simulink model "waypoint_generation_ptCloud_200802_mapdata_filtering_8m_2"  (R2020a)
settings: Solver=ode4  StartTime=0.0  StopTime=500  FixedStep=0.01  RelTol=1e-3  EnableMultiTasking=on
InitFcn:
  | detector = load('ptOPDetector.mat');
  | OPdetector = detector.OPdetector;
undefined symbols (not defined in the file): g, Kd_p, Kd_q, Kd_r, Kd_vx, Kd_vy, Kd_vz, Kff_r, Kff_vx, Kff_vy, Kff_vz, Ki_p, Ki_q, Ki_r, Ki_vx, Ki_vy, Ki_vz, Kp_p, Kp_phi, Kp_psi, Kp_q, Kp_r, Kp_theta, Kp_vx, Kp_vy, Kp_vz, M, pointCloud_center, sigma_motor, w_h
libraries: visiontextngfix x4, sharedtransform x1, shared6dof x1, simulink_extras x1
(part 2 of 3)

== matlab function waypoint_generation_ptCloud_200802_mapdata_filtering_8m_2/3D A* Algorithm/MATLAB Function2 ==
  data: current_pos input; point input; distance input; I_front_rgb input; I_back_rgb input; I_left_rgb input; I_right_rgb input; bboxes_front_raw input; openpoint_front output; bboxes_back_raw input; bboxes_left_raw input; bboxes_right_raw input; openpoint_back output; openpoint_left output; openpoint_right output; image_grid input; count output
function [openpoint_front,openpoint_back,openpoint_left,openpoint_right,count] = fcn(current_pos,point,distance,I_front_rgb,I_back_rgb,I_left_rgb,I_right_rgb,bboxes_front_raw,bboxes_back_raw,bboxes_left_raw,bboxes_right_raw,image_grid)
% function [distance_ref_front,distance_ref_back,distance_ref_left,distance_ref_right] = fcn(point,I_front_rgb,I_back_rgb,I_left_rgb,I_right_rgb,bboxes_front_raw,bboxes_back_raw,bboxes_left_raw,bboxes_right_raw)
% image_grid = 0.05;

pos_x = current_pos(1);
pos_y = current_pos(2);
pos_z = current_pos(3);

I_front = I_front_rgb(:,:,1);
I_back = I_back_rgb(:,:,1);
I_left = I_left_rgb(:,:,1);
I_right = I_right_rgb(:,:,1);

openpoint_front = nan(5,6);
openpoint_back = nan(5,6);
openpoint_left = nan(5,6);
openpoint_right = nan(5,6);
count = zeros(5,4);
thickness = distance/2;
% thickness = 2;

% bboxes_front = int16(nonzeros(bboxes_front_raw));
% bboxes_back = int16(nonzeros(bboxes_back_raw));
% bboxes_left = int16(nonzeros(bboxes_left_raw));
% bboxes_right = int16(nonzeros(bboxes_right_raw));
bboxes_front = int16(bboxes_front_raw);
bboxes_back = int16(bboxes_back_raw);
bboxes_left = int16(bboxes_left_raw);
bboxes_right = int16(bboxes_right_raw);
% distance_ref_front=[];
% distance_ref_back=[];
% distance_ref_left=[];
% distance_ref_right=[];

distance_ref_front=nan(5,1);
distance_ref_back=nan(5,1);
distance_ref_left=nan(5,1);
distance_ref_right=nan(5,1);

% aaa=1;
% if ~isempty(bboxes_front)
if ~sum(bboxes_front)==0
    for aaa = 1:numel(nonzeros(bboxes_front))/4
        if (bboxes_front(aaa,1)+bboxes_front(aaa,3)/2) >= length(I_front)/2
            distance_ref_front(aaa) = bboxes_front(aaa,1)+bboxes_front(aaa,3);
        else
            distance_ref_front(aaa) = bboxes_front(aaa,1);
        end
    end
    distance_ref_front= -(distance_ref_front - length(I_front)/2)*image_grid;           % 醫뚰몴媛?(m)
end

% if ~isempty(bboxes_back)
if ~sum(bboxes_back)==0
    for aaa = 1:numel(nonzeros(bboxes_back))/4
        if (bboxes_back(aaa,1)+bboxes_back(aaa,3)/2) >= length(I_back)/2
            distance_ref_back(aaa) = bboxes_back(aaa,1)+bboxes_back(aaa,3);
        else
            distance_ref_back(aaa) = bboxes_back(aaa,1);
        end
    end
    distance_ref_back= -(distance_ref_back - length(I_back)/2)*image_grid;              % 醫뚰몴媛?(m)
end

% if ~isempty(bboxes_left)
if ~sum(bboxes_left)==0
    for aaa = 1:numel(nonzeros(bboxes_left))/4
        if (bboxes_left(aaa,1)+bboxes_left(aaa,3)/2) >= length(I_left)/2
            distance_ref_left(aaa) = bboxes_left(aaa,1)+bboxes_left(aaa,3);
        else
            distance_ref_left(aaa) = bboxes_left(aaa,1);
        end
    end
    distance_ref_left= (distance_ref_left - length(I_left)/2)*image_grid;              % 醫뚰몴媛?(m)
end

% if ~isempty(bboxes_right)
if ~sum(bboxes_right)==0
    for aaa = 1:numel(nonzeros(bboxes_right))/4
        if (bboxes_right(aaa,1)+bboxes_right(aaa,3)/2) >= length(I_right)/2
            distance_ref_right(aaa) = bboxes_right(aaa,1)+bboxes_right(aaa,3);
        else
            distance_ref_right(aaa) = bboxes_right(aaa,1);
        end
    end
    distance_ref_right= (distance_ref_right - length(I_right)/2)*image_grid;            % 醫뚰몴媛?(m)
end

% scale = 5;
scale = 10;
distance_fb_max=-ones(length(distance_ref_front),1)*image_grid*length(I_front)/2;
distance_fb_min=ones(length(distance_ref_back),1)*image_grid*length(I_back)/2;
distance_lr_max=-ones(length(distance_ref_left),1)*image_grid*length(I_left)/2;
distance_lr_min=ones(length(distance_ref_right),1)*image_grid*length(I_right)/2;

% distance_fb_max=ones(5,1)*distance;
% distance_fb_min=-ones(5,1)*distance;
% distance_lr_max=ones(5,1)*distance;
% distance_lr_min=-ones(5,1)*distance;
    
for bbb=1:length(point)
    %     if ~isempty(distance_ref_front)
    for aaa = 1:length(distance_ref_front)
        if ~isnan(distance_ref_front(aaa))
            if point(bbb,2)>=(distance_ref_front(aaa)-image_grid*scale) && point(bbb,2)<=(distance_ref_front(aaa)+image_grid*scale)
                if point(bbb,1) > distance_fb_max(aaa)
                    distance_fb_max(aaa) = point(bbb,1);
                end
            end
        end
    end
    %     if ~isempty(distance_ref_back)
    for aaa = 1:length(distance_ref_back)
        if ~isnan(distance_ref_back(aaa))
            if point(bbb,2)>=(distance_ref_back(aaa)-image_grid*scale) && point(bbb,2)<=(distance_ref_back(aaa)+image_grid*scale)
                if point(bbb,1) < distance_fb_min(aaa)
                    distance_fb_min(aaa) = point(bbb,1);
                end
            end
        end
    end
    %     if ~isempty(distance_ref_left)
    for aaa = 1:length(distance_ref_left)
        if ~isnan(distance_ref_left(aaa))
            if point(bbb,1)>=(distance_ref_left(aaa)-image_grid*scale) && point(bbb,1)<=(distance_ref_left(aaa)+image_grid*scale)
                if point(bbb,2) > distance_lr_max(aaa)
                    distance_lr_max(aaa) = point(bbb,2);
                end
            end
        end
    end
    %     if ~isempty(distance_ref_right)
    for aaa = 1:length(distance_ref_right)
        if ~isnan(distance_ref_right(aaa))
            if point(bbb,1)>=(distance_ref_right(aaa)-image_grid*scale) && point(bbb,1)<=(distance_ref_right(aaa)+image_grid*scale)
                if point(bbb,2) < distance_lr_min(aaa)
                    distance_lr_min(aaa) = point(bbb,2);
                end
            end
        end
    end
end
bboxes_transformed_front = -(double(bboxes_front)-[ones(5,1)*length(I_front)/2, ones(5,1)*length(I_front)/2, zeros(5,1), zeros(5,1)])*image_grid;
bboxes_transformed_back = -(double(bboxes_back)-[ones(5,1)*length(I_back)/2, ones(5,1)*length(I_back)/2, zeros(5,1), zeros(5,1)])*image_grid;
bboxes_transformed_left = (double(bboxes_left)-[ones(5,1)*length(I_left)/2, ones(5,1)*length(I_left)/2, zeros(5,1), zeros(5,1)]).*[ones(5,1), -ones(5,1), ones(5,1), -ones(5,1)]*image_grid;
bboxes_transformed_right = (double(bboxes_right)-[ones(5,1)*length(I_right)/2, ones(5,1)*length(I_right)/2, zeros(5,1), zeros(5,1)]).*[ones(5,1), -ones(5,1), ones(5,1), -ones(5,1)]*image_grid;

%(x,y,z,length,width,height)
% openpoint_front = [distance_fb_max-thickness/2,bboxes_transformed_front(:,1)+bboxes_transformed_front(:,3)/2,bboxes_transformed_front(:,2)+bboxes_transformed_front(:,4)/2,thickness*ones(length(distance_fb_max),1),abs(bboxes_transformed_front(:,3)),abs(bboxes_transformed_front(:,4))];                      
% openpoint_back = [distance_fb_min+thickness/2,bboxes_transformed_back(:,1)+bboxes_transformed_back(:,3)/2,bboxes_transformed_back(:,2)+bboxes_transformed_back(:,4)/2,thickness*ones(length(distance_fb_min),1),abs(bboxes_transformed_back(:,3)),abs(bboxes_transformed_back(:,4))];
% openpoint_left = [bboxes_transformed_left(:,1)+bboxes_transformed_left(:,3)/2 , distance_lr_max-thickness/2 , bboxes_transformed_left(:,2)+bboxes_transformed_left(:,4)/2,abs(bboxes_transformed_left(:,3)),thickness*ones(length(distance_lr_max),1),abs(bboxes_transformed_left(:,4))];
% openpoint_right = [bboxes_transformed_right(:,1)+bboxes_transformed_right(:,3)/2 , distance_lr_min+thickness/2 , bboxes_transformed_right(:,2)+bboxes_transformed_right(:,4)/2,abs(bboxes_transformed_right(:,3)),thickness*ones(length(distance_lr_min),1),abs(bboxes_transformed_right(:,4))];

for aaa = 1 : 5
    if ~(distance_fb_max(aaa) == -image_grid*length(I_front)/2)
        openpoint_front(aaa,:) = [distance_fb_max(aaa)-thickness/2 , bboxes_transformed_front(aaa,1)+bboxes_transformed_front(aaa,3)/2+pos_y , bboxes_transformed_front(aaa,2)+bboxes_transformed_front(aaa,4)/2+pos_z , thickness , abs(bboxes_transformed_front(aaa,3)) , abs(bboxes_transformed_front(aaa,4))];
%         openpoint_front(aaa,:) = [distance_fb_max(aaa)-thickness/2+pos_x , bboxes_transformed_front(aaa,1)+bboxes_transformed_front(aaa,3)/2+pos_y , bboxes_transformed_front(aaa,2)+bboxes_transformed_front(aaa,4)/2+pos_z , thickness , abs(bboxes_transformed_front(aaa,3)) , abs(bboxes_transformed_front(aaa,4))];
    end
    if ~(distance_fb_min(aaa) == image_grid*length(I_front)/2)
        openpoint_back(aaa,:) = [distance_fb_min(aaa)+thickness/2 , bboxes_transformed_back(aaa,1)+bboxes_transformed_back(aaa,3)/2+pos_y , bboxes_transformed_back(aaa,2)+bboxes_transformed_back(aaa,4)/2+pos_z , thickness , abs(bboxes_transformed_back(aaa,3)) , abs(bboxes_transformed_back(aaa,4))];
%         openpoint_back(aaa,:) = [distance_fb_min(aaa)+thickness/2+pos_x , bboxes_transformed_back(aaa,1)+bboxes_transformed_back(aaa,3)/2+pos_y , bboxes_transformed_back(aaa,2)+bboxes_transformed_back(aaa,4)/2+pos_z , thickness , abs(bboxes_transformed_back(aaa,3)) , abs(bboxes_transformed_back(aaa,4))];
    end
    if ~(distance_lr_max(aaa) == -image_grid*length(I_front)/2)
        openpoint_left(aaa,:) = [bboxes_transformed_left(aaa,1)+bboxes_transformed_left(aaa,3)/2+pos_x , distance_lr_max(aaa)-thickness/2 , bboxes_transformed_left(aaa,2)+bboxes_transformed_left(aaa,4)/2+pos_z , abs(bboxes_transformed_left(aaa,3)) , thickness , abs(bboxes_transformed_left(aaa,4))];
%         openpoint_left(aaa,:) = [bboxes_transformed_left(aaa,1)+bboxes_transformed_left(aaa,3)/2+pos_x , distance_lr_max(aaa)-thickness/2+pos_y , bboxes_transformed_left(aaa,2)+bboxes_transformed_left(aaa,4)/2+pos_z , abs(bboxes_transformed_left(aaa,3)) , thickness , abs(bboxes_transformed_left(aaa,4))];
    end
    if ~(distance_lr_min(aaa) == image_grid*length(I_front)/2)
        openpoint_right(aaa,:) = [bboxes_transformed_right(aaa,1)+bboxes_transformed_right(aaa,3)/2+pos_x , distance_lr_min(aaa)+thickness/2 , bboxes_transformed_right(aaa,2)+bboxes_transformed_right(aaa,4)/2+pos_z , abs(bboxes_transformed_right(aaa,3)) , thickness , abs(bboxes_transformed_right(aaa,4))];
%         openpoint_right(aaa,:) = [bboxes_transformed_right(aaa,1)+bboxes_transformed_right(aaa,3)/2+pos_x , distance_lr_min(aaa)+thickness/2+pos_y , bboxes_transformed_right(aaa,2)+bboxes_transformed_right(aaa,4)/2+pos_z , abs(bboxes_transformed_right(aaa,3)) , thickness , abs(bboxes_transformed_right(aaa,4))];
    end
end

for aaa = 1:5
    count_front = 0;
    count_back = 0;
    count_left = 0;
    count_right = 0;
    obstacle_check_front = 0;
    obstacle_check_back = 0;
    obstacle_check_left = 0;
    obstacle_check_right = 0;
    for bbb = 1:length(point)
        if ((point(bbb,1) > openpoint_front(aaa,1)-thickness/10) && (point(bbb,1) < openpoint_front(aaa,1)+thickness/10)) && (point(bbb,2) > openpoint_front(aaa,2)-thickness/10) && (point(bbb,2) < openpoint_front(aaa,2)+thickness/10)
%         if ((point(bbb,1) > openpoint_front(aaa,1)-thickness/2-thickness/10) && (point(bbb,1) < openpoint_front(aaa,1)-thickness/2+thickness/10)) && (point(bbb,2) > openpoint_front(aaa,2)-thickness/10) && (point(bbb,2) < openpoint_front(aaa,2)+thickness/10)
            count_front = count_front+1;
        end
        if ((point(bbb,1) > openpoint_back(aaa,1)-thickness/10) && (point(bbb,1) < openpoint_back(aaa,1)+thickness/10)) && (point(bbb,2) > openpoint_back(aaa,2)-thickness/10) && (point(bbb,2) < openpoint_back(aaa,2)+thickness/10)
%         if ((point(bbb,1) > openpoint_back(aaa,1)+thickness/2-thickness/10) && (point(bbb,1) < openpoint_back(aaa,1)+thickness/2+thickness/10)) && (point(bbb,2) > openpoint_back(aaa,2)-thickness/10) && (point(bbb,2) < openpoint_back(aaa,2)+thickness/10)
            count_back = count_back+1;
        end
        if ((point(bbb,1) > openpoint_left(aaa,1)-thickness/10) && (point(bbb,1) < openpoint_left(aaa,1)+thickness/10)) && (point(bbb,2) > openpoint_left(aaa,2)-thickness/10) && (point(bbb,2) < openpoint_left(aaa,2)+thickness/10)
%         if ((point(bbb,1) > openpoint_left(aaa,1)-thickness/10) && (point(bbb,1) < openpoint_left(aaa,1)+thickness/10)) && (point(bbb,2) > openpoint_left(aaa,2)-thickness/2-thickness/10) && (point(bbb,2) < openpoint_left(aaa,2)-thickness/2+thickness/10)
            count_left = count_left+1;
        end
        if ((point(bbb,1) > openpoint_right(aaa,1)-thickness/10) && (point(bbb,1) < openpoint_right(aaa,1)+thickness/10)) && (point(bbb,2) > openpoint_right(aaa,2)-thickness/10) && (point(bbb,2) < openpoint_right(aaa,2)+thickness/10)
%         if ((point(bbb,1) > openpoint_right(aaa,1)-thickness/10) && (point(bbb,1) < openpoint_right(aaa,1)+thickness/10)) && (point(bbb,2) > openpoint_right(aaa,2)+thickness/2-thickness/10) && (point(bbb,2) < openpoint_right(aaa,2)+thickness/2+thickness/10)
            count_right= count_right+1;
        end
        
        if ((point(bbb,1) > openpoint_front(aaa,1)-1) && (point(bbb,1) < openpoint_front(aaa,1)+1)) && ((point(bbb,2) > openpoint_front(aaa,2)-1) && (point(bbb,2) < openpoint_front(aaa,2)+1)) && ((point(bbb,3) > openpoint_front(aaa,3)-0.5) && (point(bbb,3) < openpoint_front(aaa,3)+0.5))
            obstacle_check_front = obstacle_check_front+1;
        end
        if ((point(bbb,1) > openpoint_back(aaa,1)-1) && (point(bbb,1) < openpoint_back(aaa,1)+1)) && ((point(bbb,2) > openpoint_back(aaa,2)-1) && (point(bbb,2) < openpoint_back(aaa,2)+1)) && ((point(bbb,3) > openpoint_back(aaa,3)-0.5) && (point(bbb,3) < openpoint_back(aaa,3)+0.5))
            obstacle_check_back = obstacle_check_back+1;
        end
        if ((point(bbb,1) > openpoint_left(aaa,1)-1) && (point(bbb,1) < openpoint_left(aaa,1)+1)) && ((point(bbb,2) > openpoint_left(aaa,2)-1) && (point(bbb,2) < openpoint_left(aaa,2)+1)) && ((point(bbb,3) > openpoint_left(aaa,3)-0.5) && (point(bbb,3) < openpoint_left(aaa,3)+0.5))
            obstacle_check_left = obstacle_check_left+1;
        end
        if ((point(bbb,1) > openpoint_right(aaa,1)-1) && (point(bbb,1) < openpoint_right(aaa,1)+1)) && ((point(bbb,2) > openpoint_right(aaa,2)-1) && (point(bbb,2) < openpoint_right(aaa,2)+1)) && ((point(bbb,3) > openpoint_right(aaa,3)-0.5) && (point(bbb,3) < openpoint_right(aaa,3)+0.5))
            obstacle_check_right= obstacle_check_right+1;
        end
        
    end
    %유효성 체크
    count(aaa,:) = [count_front, count_back, count_left, count_right];
    if count_front < 2 || obstacle_check_front > 0
%     if obstacle_check_front > 0
        openpoint_front(aaa,:) = nan(1,6);
    end
    if count_back< 2 || obstacle_check_back > 0
%     if obstacle_check_back > 0
        openpoint_back(aaa,:) = nan(1,6);
    end
    if count_left< 2 || obstacle_check_left > 0
%     if obstacle_check_left > 0
        openpoint_left(aaa,:) = nan(1,6);
    end
    if count_right< 2 || obstacle_check_right > 0
%     if obstacle_check_right > 0
        openpoint_right(aaa,:) = nan(1,6);
    end
end

== matlab function waypoint_generation_ptCloud_200802_mapdata_filtering_8m_2/3D A* Algorithm/MATLAB Function3 ==
  data: Image input; Image_resized output; detector_image_size input
function Image_resized = fcn(Image,detector_image_size)
Image_resized = imresize(Image,[400 400]);

== matlab function waypoint_generation_ptCloud_200802_mapdata_filtering_8m_2/3D A* Algorithm/MATLAB Function4 ==
  data: Image input; Image_resized output; detector_image_size input
function Image_resized = fcn(Image,detector_image_size)
Image_resized = imresize(Image,[400 400]);

== matlab function waypoint_generation_ptCloud_200802_mapdata_filtering_8m_2/3D A* Algorithm/MATLAB Function5 ==
  data: Image input; Image_resized output; detector_image_size input
function Image_resized = fcn(Image,detector_image_size)
Image_resized = imresize(Image,[400 400]);

== matlab function waypoint_generation_ptCloud_200802_mapdata_filtering_8m_2/3D A* Algorithm/MATLAB Function11 ==
  settings: updateMethod=DISCRETE
  data: pos_grid input; waypoint_given input; point_cmd output; waypoint_gen input; auto_flag output; waypoint_set output; Obstacle input
function [point_cmd,auto_flag,waypoint_set] = gen_waypoint(pos_grid,waypoint_given,waypoint_gen,Obstacle)

persistent flag autonomous_mode_flag waypoint_old waypoint_pre

if isempty(flag)
    flag = 1;
end
if isempty(autonomous_mode_flag)
    autonomous_mode_flag = 0;
end
if isempty(waypoint_old)
    waypoint_old = nan(20,3);
end
if isempty(waypoint_pre)
    waypoint_pre = nan(20,3);
    for aaa = 1:numel(waypoint_given)/3
        waypoint_pre(aaa,:)=waypoint_given(aaa,:);
    end
end
% if isempty(explor_grid)
%     explor_grid = zeros(30,20,6);
% end
% grid_explor_size = 1;
% explor_map_init = [15, 10, 3];
pos_grid = int32(pos_grid);
% pos_explor_grid = int32(pos_cur'./grid_explor_size+explor_map_size);
% pos_explor_grid = int32([pos_cur(1)/grid_explor_size+explor_map_init(1), pos_cur(2)/grid_explor_size+explor_map_init(2) , pos_cur(3)/grid_explor_size+explor_map_init(3)]);

% waypoint_gen_grid = waypoint_gen ./ 1 15,10,3;
% % 중복성 체크
% explor_grid(pos_explor_grid(1),pos_explor_grid(2),pos_explor_grid(3))=1;
% for abc=1:numel(waypoint_gen)/3
%     if ~isnan(waypoint_gen(abc,1)) && ~isnan(waypoint_gen(abc,2)) && ~isnan(waypoint_gen(abc,3))
%         if explor_grid(int32(waypoint_gen(abc,1)+explor_map_init(1)),int32(waypoint_gen(abc,2)+explor_map_init(2)),int32(waypoint_gen(abc,3)+explor_map_init(3))) == 1
%             waypoint_gen(abc,:) = nan(1,3);
%         end
%     end
% end


waypoint_pre_x = waypoint_pre(:,1);
waypoint_pre_y = waypoint_pre(:,2);
waypoint_pre_z = waypoint_pre(:,3);

point_cmd_temp = int32([waypoint_pre_x(flag) waypoint_pre_y(flag) waypoint_pre_z(flag)]);
waypoint_auto_set = nan(40,3);
waypoint_auto_set_sorted = nan(40,3);
waypoint_distance = nan(40,1);

for lll = 1:numel(waypoint_gen)/3
    if ~isnan(waypoint_gen(lll,1)) && ~isnan(waypoint_gen(lll,2)) && ~isnan(waypoint_gen(lll,3))
%         if waypoint_gen(lll,1)>0 && waypoint_gen(lll,2)>0 && waypoint_gen(lll,3)>0
            if Obstacle(waypoint_gen(lll,1),waypoint_gen(lll,2),waypoint_gen(lll,3)) == 1
                waypoint_gen(lll,:)=nan(1,3);
            end
%         end
    end
end


if autonomous_mode_flag==0
    if abs(point_cmd_temp(1)-pos_grid(1)) <= 0 && abs(point_cmd_temp(2)-pos_grid(2)) <= 0 && abs(point_cmd_temp(3)-pos_grid(3)) <= 0
        flag = flag + 1;
        
        if flag == numel(rmmissing(waypoint_pre))/3 + 1
            flag = numel(rmmissing(waypoint_pre))/3;
            autonomous_mode_flag = 1;
        end
    end
    
    % waypoint_gen_filtered = rmmissing(waypoint_gen);
    % if ~isempty(waypoint_gen_filtered)
    %     if flag == numel(waypoint_pre)/3
    %         waypoint_x = waypoint_gen_filtered(1,1);
    %         waypoint_y = waypoint_gen_filtered(1,2);
    %         waypoint_z = waypoint_gen_filtered(1,3);
    %     end
    % end
elseif autonomous_mode_flag==1
    waypoint_auto_old = rmmissing(waypoint_old);
    waypoint_auto_new = rmmissing(waypoint_gen);
    if isempty(waypoint_auto_old)
        waypoint_auto_old = waypoint_auto_new;
    end
    
    if ~isempty(waypoint_auto_old) && ~isempty(waypoint_auto_new)
        for mmm = numel(waypoint_auto_new)/3:-1:1
            changed_flag=0;
            for nnn = 1:numel(waypoint_auto_old)/3
                if ((waypoint_auto_new(mmm,1)-waypoint_auto_old(nnn,1))^2+(waypoint_auto_new(mmm,2)-waypoint_auto_old(nnn,2))^2+(waypoint_auto_new(mmm,3)-waypoint_auto_old(nnn,3))^2)<100
                    waypoint_auto_old(nnn,:)=waypoint_auto_new(mmm,:);
                    changed_flag=1;
                end
            end
            if changed_flag == 1
                waypoint_auto_new(mmm,:)=nan(1,3);
            end
        end
%         waypoint_auto_set_temp = cat(1,unique(waypoint_auto_old,'stable','rows'),waypoint_auto_new);

%             waypoint_auto_set_temp = rmmissing(cat(1,waypoint_auto_new,unique(waypoint_auto_old,'stable','rows')));
            waypoint_auto_set_temp = rmmissing(cat(1,unique(waypoint_auto_old,'stable','rows'),waypoint_auto_new));

        
        for aaa = 1:numel(waypoint_auto_set_temp)/3
            waypoint_auto_set(aaa,:)=waypoint_auto_set_temp(aaa,:);
            waypoint_distance(aaa) = (((waypoint_auto_set(aaa,1)-pos_grid(1))^2+(waypoint_auto_set(aaa,2)-pos_grid(2))^2+(waypoint_auto_set(aaa,3)-pos_grid(3))^2));
        end
        [~,waypoint_index]=sort(waypoint_distance);
        
        for aaa = 1:length(waypoint_index)
            waypoint_auto_set_sorted(aaa,:)=waypoint_auto_set(waypoint_index(aaa),:);
        end
%         waypoint_auto_set(1:aaa,:)=waypoint_auto_set_temp(waypoint_index,:);
        
        point_cmd_temp = int32([waypoint_auto_set_sorted(1,1), waypoint_auto_set_sorted(1,2), waypoint_auto_set_sorted(1,3)]);
        
        if abs(point_cmd_temp(1)-pos_grid(1)) <= 0 && abs(point_cmd_temp(2)-pos_grid(2)) <= 0 && abs(point_cmd_temp(3)-pos_grid(3)) <= 0
            waypoint_auto_set_sorted = [waypoint_auto_set_sorted(2:end,:); nan(1,3)];            
        end
        
        waypoint_old = waypoint_auto_set_sorted(1:20,:);
        
        
    else
        if ~isnan(waypoint_old(1,1)) && ~isnan(waypoint_old(1,2)) && ~isnan(waypoint_old(1,3))
            point_cmd_temp = int32([waypoint_old(1,1), waypoint_old(1,2), waypoint_old(1,3)]);
%             waypoint_pre = waypoint_old;
%             autonomous_mode_flag = 0;
%             flag = 1;

            if abs(point_cmd_temp(1)-pos_grid(1)) <= 0 && abs(point_cmd_temp(2)-pos_grid(2)) <= 0 && abs(point_cmd_temp(3)-pos_grid(3)) <= 0
                waypoint_old = [waypoint_old(2:end,:); nan(1,3)];            
            end


        else
            point_cmd_temp = int32([pos_grid(1), pos_grid(2), pos_grid(3)]);
        end
    end
end


% point_cmd = int32([waypoint_pre_x(flag) waypoint_pre_y(flag) waypoint_pre_z(flag)]);
point_cmd = point_cmd_temp;


auto_flag = autonomous_mode_flag;
waypoint_set = waypoint_auto_set_sorted;


end

== matlab function waypoint_generation_ptCloud_200802_mapdata_filtering_8m_2/3D A* Algorithm/MATLAB Function12 ==
  data: odom_input input; pos_grid output; pos_init input
function pos_grid = odom_grid(odom_input,pos_init)

odom = zeros(1,3);
odom(1,1) = odom_input(1);
odom(1,2) = odom_input(2);
odom(1,3) = odom_input(3);

start_point = [pos_init(1) pos_init(2) pos_init(3)];

% pos_x = int16(odom(1)/0.2+0.5);
% pos_y = int16(odom(2)/0.2+0.5);
% pos_z = int16(odom(3)/0.2+0.5);
pos_x = int16(odom(1)/0.2);
pos_y = int16(odom(2)/0.2);
pos_z = int16(odom(3)/0.2);

pos_grid = [pos_x+start_point(1) pos_y+start_point(2) pos_z+start_point(3)];

end

== matlab function waypoint_generation_ptCloud_200802_mapdata_filtering_8m_2/3D A* Algorithm/MATLAB Function6 ==
  settings: updateMethod=DISCRETE
  data: pos_cur input; distance input; pos_init input; openpoint_front input; waypoint_gen output; openpoint_back input; openpoint_left input; openpoint_right input; pos_explor_grid output
function [waypoint_gen,pos_explor_grid] = fcn(pos_cur,distance,pos_init,openpoint_front,openpoint_back,openpoint_left,openpoint_right)

persistent explor_grid

if isempty(explor_grid)
    explor_grid = zeros(50,50,10);
end
% grid_explor_size = 4;
grid_explor_size = distance/2;
grid_size = 0.2;
explor_map_init = [25, 25, 5];
pos_explor_grid = int32([pos_cur(1)/grid_explor_size+explor_map_init(1), pos_cur(2)/grid_explor_size+explor_map_init(2) , pos_cur(3)/grid_explor_size+explor_map_init(3)]);

explor_grid(pos_explor_grid(1),pos_explor_grid(2),pos_explor_grid(3))=1;



for abc=1:numel(openpoint_front)/6
    if ~isnan(openpoint_front(abc,1)) && ~isnan(openpoint_front(abc,2)) && ~isnan(openpoint_front(abc,3))
        if explor_grid(int16(openpoint_front(abc,1)/grid_explor_size+explor_map_init(1)),int16(openpoint_front(abc,2)/grid_explor_size+explor_map_init(2)),int16(openpoint_front(abc,3)/grid_explor_size+explor_map_init(3))) == 1
            openpoint_front(abc,:) = nan(1,6);
        end
    end
end
for abc=1:numel(openpoint_back)/6
    if ~isnan(openpoint_back(abc,1)) && ~isnan(openpoint_back(abc,2)) && ~isnan(openpoint_back(abc,3))
        if explor_grid(int16(openpoint_back(abc,1)/grid_explor_size+explor_map_init(1)),int16(openpoint_back(abc,2)/grid_explor_size+explor_map_init(2)),int16(openpoint_back(abc,3)/grid_explor_size+explor_map_init(3))) == 1
            openpoint_back(abc,:) = nan(1,6);
        end
    end
end
for abc=1:numel(openpoint_left)/6
    if ~isnan(openpoint_left(abc,1)) && ~isnan(openpoint_left(abc,2)) && ~isnan(openpoint_left(abc,3))
        if explor_grid(int16(openpoint_left(abc,1)/grid_explor_size+explor_map_init(1)),int16(openpoint_left(abc,2)/grid_explor_size+explor_map_init(2)),int16(openpoint_left(abc,3)/grid_explor_size+explor_map_init(3))) == 1
            openpoint_left(abc,:) = nan(1,6);
        end
    end
end
for abc=1:numel(openpoint_right)/6
    if ~isnan(openpoint_right(abc,1)) && ~isnan(openpoint_right(abc,2)) && ~isnan(openpoint_right(abc,3))
        if explor_grid(int16(openpoint_right(abc,1)/grid_explor_size+explor_map_init(1)),int16(openpoint_right(abc,2)/grid_explor_size+explor_map_init(2)),int16(openpoint_right(abc,3)/grid_explor_size+explor_map_init(3))) == 1
            openpoint_right(abc,:) = nan(1,6);
        end
    end
end



openpoint_front_grid = int16(openpoint_front/grid_size);
openpoint_back_grid = int16(openpoint_back/grid_size);
openpoint_left_grid = int16(openpoint_left/grid_size);
openpoint_right_grid = int16(openpoint_right/grid_size);



waypoint_gen_front = nan(5,3);
waypoint_gen_back = nan(5,3);
waypoint_gen_left = nan(5,3);
waypoint_gen_right = nan(5,3);

for aaa = 1:5
    if ~isnan(openpoint_front(aaa,1))
        waypoint_gen_front(aaa,:) = [openpoint_front_grid(aaa,1)+int16(pos_init(1)), openpoint_front_grid(aaa,2)+int16(pos_init(2)), openpoint_front_grid(aaa,3)+int16(pos_init(3))];
    end
    if ~isnan(openpoint_back(aaa,1))
        waypoint_gen_back(aaa,:) = [openpoint_back_grid(aaa,1)+int16(pos_init(1)), openpoint_back_grid(aaa,2)+int16(pos_init(2)), openpoint_back_grid(aaa,3)+int16(pos_init(3))];
    end
    if ~isnan(openpoint_left(aaa,1))
        waypoint_gen_left(aaa,:) = [openpoint_left_grid(aaa,1)+int16(pos_init(1)), openpoint_left_grid(aaa,2)+int16(pos_init(2)), openpoint_left_grid(aaa,3)+int16(pos_init(3))];
    end
    if ~isnan(openpoint_right(aaa,1))
        waypoint_gen_right(aaa,:) = [openpoint_right_grid(aaa,1)+int16(pos_init(1)), openpoint_right_grid(aaa,2)+int16(pos_init(2)), openpoint_right_grid(aaa,3)+int16(pos_init(3))];
    end
end

waypoint_gen = [waypoint_gen_front;waypoint_gen_back;waypoint_gen_left;waypoint_gen_right];

== matlab function waypoint_generation_ptCloud_200802_mapdata_filtering_8m_2/3D A* Algorithm/MATLAB Function9 ==
  data: bboxes_raw input; bboxes output; bboxes_size input
function bboxes = fcn(bboxes_raw,bboxes_size)
bboxes = zeros(5,4);
% bboxes_nonzeros = nonzeros(bboxes_raw);
% num_bboxes = min(numel(bboxes_nonzeros)/4,5);
num_bboxes = bboxes_size(1);

if num_bboxes>0 && num_bboxes<6
    for aaa = 1:num_bboxes
        bboxes(aaa,:) = [bboxes_raw(aaa+0*num_bboxes),bboxes_raw(aaa+1*num_bboxes),bboxes_raw(aaa+2*num_bboxes),bboxes_raw(aaa+3*num_bboxes)];
%         bboxes(aaa,:) = [bboxes_nonzeros(aaa+0*num_bboxes),bboxes_nonzeros(aaa+1*num_bboxes),bboxes_nonzeros(aaa+2*num_bboxes),bboxes_nonzeros(aaa+3*num_bboxes)];
    end
end
% bboxes(1:num_bboxes,:) = reshape(bboxes_nonzeros,num_bboxes,4);

== matlab function waypoint_generation_ptCloud_200802_mapdata_filtering_8m_2/3D A* Algorithm/MATLAB Function10 ==
  data: bboxes_raw input; bboxes output; bboxes_size input
function bboxes = fcn(bboxes_raw,bboxes_size)
bboxes = zeros(5,4);
% bboxes_nonzeros = nonzeros(bboxes_raw);
% num_bboxes = min(numel(bboxes_nonzeros)/4,5);
num_bboxes = bboxes_size(1);

if num_bboxes>0 && num_bboxes<6
    for aaa = 1:num_bboxes
        bboxes(aaa,:) = [bboxes_raw(aaa+0*num_bboxes),bboxes_raw(aaa+1*num_bboxes),bboxes_raw(aaa+2*num_bboxes),bboxes_raw(aaa+3*num_bboxes)];
%         bboxes(aaa,:) = [bboxes_nonzeros(aaa+0*num_bboxes),bboxes_nonzeros(aaa+1*num_bboxes),bboxes_nonzeros(aaa+2*num_bboxes),bboxes_nonzeros(aaa+3*num_bboxes)];
    end
end
% bboxes(1:num_bboxes,:) = reshape(bboxes_nonzeros,num_bboxes,4);

== matlab function waypoint_generation_ptCloud_200802_mapdata_filtering_8m_2/Generation_Angle_error/Attitude Generation (phi,theta,psi) ==
  data: DCM input; acc_cmd input; angle_error output; R_rp_x output
function [angle_error,R_rp_x]  = fcn(DCM,acc_cmd)
%#codegen

R_z           = DCM(3,:)'; 

% for i = 1:length(R_z)
%     if abs(R_z(i)) < 0.001
%         R_z(i) = 0;
%     end
% end

acc_unit      = R_z     / norm(R_z);
acc_cmd_unit  = acc_cmd / norm(acc_cmd);

angle_error = DCM * cross(acc_unit,acc_cmd_unit); %% e_R , consider phi, theta


% Calculate R_rp_x
angle = atan(norm(cross(acc_unit,acc_cmd_unit))/norm(dot(acc_unit,acc_cmd_unit))); % only phi,theta

e_R = angle_error;
R= DCM';

% e_R_cp matrix cross product
e_R_cp = zeros(3,3);
e_R_cp(1,2) = -e_R(3);
e_R_cp(1,3) =  e_R(2);
e_R_cp(2,1) =  e_R(3);
e_R_cp(2,3) = -e_R(1);
e_R_cp(3,1) = -e_R(2);
e_R_cp(3,2) =  e_R(1);

% Result
R_rp = R*(eye(3,3) + e_R_cp*sin(angle) + e_R_cp*e_R_cp*(1-cos(angle)));
R_rp_x = R_rp(:,1);
% acc_cmd_result = R_rp(:,3);

== matlab function waypoint_generation_ptCloud_200802_mapdata_filtering_8m_2/3D A* Algorithm/MATLAB Function13 ==
  data: bboxes_raw input; bboxes output; bboxes_size input
function bboxes = fcn(bboxes_raw,bboxes_size)
bboxes = zeros(5,4);
% bboxes_nonzeros = nonzeros(bboxes_raw);
% num_bboxes = min(numel(bboxes_nonzeros)/4,5);
num_bboxes = bboxes_size(1);

if num_bboxes>0 && num_bboxes<6
    for aaa = 1:num_bboxes
        bboxes(aaa,:) = [bboxes_raw(aaa+0*num_bboxes),bboxes_raw(aaa+1*num_bboxes),bboxes_raw(aaa+2*num_bboxes),bboxes_raw(aaa+3*num_bboxes)];
%         bboxes(aaa,:) = [bboxes_nonzeros(aaa+0*num_bboxes),bboxes_nonzeros(aaa+1*num_bboxes),bboxes_nonzeros(aaa+2*num_bboxes),bboxes_nonzeros(aaa+3*num_bboxes)];
    end
end
% bboxes(1:num_bboxes,:) = reshape(bboxes_nonzeros,num_bboxes,4);

== matlab function waypoint_generation_ptCloud_200802_mapdata_filtering_8m_2/3D A* Algorithm/MATLAB Function14 ==
  data: bboxes_raw input; bboxes output; bboxes_size input
function bboxes = fcn(bboxes_raw,bboxes_size)
bboxes = zeros(5,4);
% bboxes_nonzeros = nonzeros(bboxes_raw);
% num_bboxes = min(numel(bboxes_nonzeros)/4,5);
num_bboxes = bboxes_size(1);

if num_bboxes>0 && num_bboxes<6
    for aaa = 1:num_bboxes
        bboxes(aaa,:) = [bboxes_raw(aaa+0*num_bboxes),bboxes_raw(aaa+1*num_bboxes),bboxes_raw(aaa+2*num_bboxes),bboxes_raw(aaa+3*num_bboxes)];
%         bboxes(aaa,:) = [bboxes_nonzeros(aaa+0*num_bboxes),bboxes_nonzeros(aaa+1*num_bboxes),bboxes_nonzeros(aaa+2*num_bboxes),bboxes_nonzeros(aaa+3*num_bboxes)];
    end
end
% bboxes(1:num_bboxes,:) = reshape(bboxes_nonzeros,num_bboxes,4);

== matlab function waypoint_generation_ptCloud_200802_mapdata_filtering_8m_2/3D A* Algorithm/MATLAB Function7 ==
  settings: updateMethod=DISCRETE
  data: pos_current input; optimal_path_x output size=[128 1]; point_cmd input; Obstacle input; pos_init input; optimal_path_y output size=[128 1]; optimal_path_z output size=[128 1]
function [optimal_path_x,optimal_path_y,optimal_path_z] = Astar_algorithm_function(pos_current,point_cmd,Obstacle,pos_init)

persistent optimal sample

if isempty(optimal)
    optimal = nan(128,3);
    sample = 99;
%     sample = 19;
end


sample = sample + 1;

if sample == 100
% if sample == 20
    sample = 1;
    
    mapsize = [150 150 30];
    
    Height = mapsize(1);        % x
    Width = mapsize(2);         % y
    Alt = mapsize(3);            % z
    
    Start = pos_current;
    Goal = point_cmd;
    look = 2;
    H_weight = 1.2;
    
    G_cost = zeros(2*look+1,2*look+1,2*look+1);
    for i = 1:2*look+1
        for j = 1:2*look+1
            for k = 1:2*look+1
                temp = [look+1 look+1 look+1]-[i j k];
                G_cost(i,j,k) = (min(sqrt(sum(abs(temp).^2,2))));
            end
        end
    end
    
    G_top2 = G_cost(:,:,1);
    G_top1 = G_cost(:,:,2);
    G_mid = G_cost(:,:,3);
    G_bottom1 = G_cost(:,:,4);
    G_bottom2 = G_cost(:,:,5);
    
    
    GScore = inf(Height,Width,Alt);
    GScore_temp = zeros(2*look+1,2*look+1,2*look+1);
    HScore = zeros(Height,Width,Alt);
    FScore = inf(Height,Width,Alt);
    ClosedMAT = zeros(Height,Width,Alt);
    CX = int32(Start(1));
    CY = int32(Start(2));
    CZ = int32(Start(3));
    ParentX = inf(Height,Width,Alt);
    ParentY = inf(Height,Width,Alt);
    ParentZ = inf(Height,Width,Alt);
    ParentX(CX,CY,CZ) = CX;
    ParentY(CX,CY,CZ) = CY;
    ParentZ(CX,CY,CZ) = CZ;
    
    %%%%%%%%%%%%%%%% Define Heuristic %%%%%%%%%%%%%%%%%%%%%%%
    for k=1:Alt
        for j=1:Width
            for i=1:Height
                
                temp = (int32(Goal) - int32([i j k])) ;
                Distance=(min(sqrt(sum(abs(temp).^2,2))));
                HScore(i,j,k)=Distance*H_weight;               % (1+sqrt(2))/sqrt(3)
                
            end
        end
    end
    
    FScore(Start(1),Start(2),Start(3)) = HScore(Start(1),Start(2),Start(3));
    GScore(Start(1),Start(2),Start(3)) = 0;
    ClosedMAT(Obstacle==1)=1;
    REACHGOAL = 0;
    
    while 1
        
        MinFScore = min(min(min(FScore)));         % Find Minimun FScore
        if isinf(MinFScore)
            disp('Fail');
            break
        end
        
        
        [minF_x,minF_y] = find(FScore==MinFScore);
        HScore_temp = inf(1,10);
        
        minHScore = 1;
        for i = 1:length(minF_x)
            Current_pose_temp = [minF_x(i) rem(minF_y(i),Width) fix(minF_y(i)/Width)+1];     % H가 가장 적은걸로 먼저 선택
            CX_temp=Current_pose_temp(1);
            CY_temp=Current_pose_temp(2);
            CZ_temp=Current_pose_temp(3);
            HScore_temp(i) = HScore(CX_temp,CY_temp,CZ_temp);
            minHScore = find(HScore_temp == min(HScore_temp));
        end
        
        
        Current_pose = int32([minF_x(minHScore(1)) rem(minF_y(minHScore(1)),Width) fix(minF_y(minHScore(1))/Width)+1]);     % H가 가장 적은걸로 먼저 선택
        CX=Current_pose(1);
        CY=Current_pose(2);
        CZ=Current_pose(3);
        
        
        
        GScore_temp(:,:,1) = GScore(CX,CY,CZ) + G_top2;
        GScore_temp(:,:,2) = GScore(CX,CY,CZ) + G_top1;
        GScore_temp(:,:,3) = GScore(CX,CY,CZ) + G_mid;
        GScore_temp(:,:,4) = GScore(CX,CY,CZ) + G_bottom1;
        GScore_temp(:,:,5) = GScore(CX,CY,CZ) + G_bottom2;
        
        
        
        
        %%%%%%%%%%%%% GScore update %%%%%%%%%%%%%
        
        GScore(CX-look:CX+look,CY-look:CY+look,CZ+2) = min(GScore_temp(:,:,1),GScore(CX-look:CX+look,CY-look:CY+look,CZ+2)) ;
        GScore(CX-look:CX+look,CY-look:CY+look,CZ+1) = min(GScore_temp(:,:,2),GScore(CX-look:CX+look,CY-look:CY+look,CZ+1));
        GScore(CX-look:CX+look,CY-look:CY+look,CZ) = min(GScore_temp(:,:,3), GScore(CX-look:CX+look,CY-look:CY+look,CZ));
        GScore(CX-look:CX+look,CY-look:CY+look,CZ-1) = min(GScore_temp(:,:,4),GScore(CX-look:CX+look,CY-look:CY+look,CZ-1));
        GScore(CX-look:CX+look,CY-look:CY+look,CZ-2) = min(GScore_temp(:,:,5),GScore(CX-look:CX+look,CY-look:CY+look,CZ-2));
        
        
        FScore = GScore + HScore;
        %     ClosedMAT(CX,CY,CZ) = 1;
        ClosedMAT(CX-(look-1):CX+(look-1),CY-(look-1):CY+(look-1),CZ-(look-1):CZ+(look-1)) = 1;
        FScore(ClosedMAT==1) = inf;
        %     Check_FScore = FScore(CX-look:CX+look,CY-look:CY+look,CZ-look:CZ+look);
        
        
        
        [G_row1,G_col1] = find( GScore(CX-look:CX+look,CY-look:CY+look,CZ+2) == GScore_temp(:,:,1) );
        [G_row2,G_col2] = find( GScore(CX-look:CX+look,CY-look:CY+look,CZ+1) == GScore_temp(:,:,2) );
        [G_row3,G_col3] = find( GScore(CX-look:CX+look,CY-look:CY+look,CZ) == GScore_temp(:,:,3) );
        [G_row4,G_col4] = find( GScore(CX-look:CX+look,CY-look:CY+look,CZ-1) == GScore_temp(:,:,4) );
        [G_row5,G_col5] = find( GScore(CX-look:CX+look,CY-look:CY+look,CZ-2) == GScore_temp(:,:,5) );
        
        
        G_row1 = int32(G_row1);
        G_row2 = int32(G_row2);
        G_row3 = int32(G_row3);
        G_row4 = int32(G_row4);
        G_row5 = int32(G_row5);
        
        G_col1 = int32(G_col1);
        G_col2 = int32(G_col2);
        G_col3 = int32(G_col3);
        G_col4 = int32(G_col4);
        G_col5 = int32(G_col5);
        
        G_row1 = G_row1+CX-(look+1);
        G_row2 = G_row2+CX-(look+1);
        G_row3 = G_row3+CX-(look+1);
        G_row4 = G_row4+CX-(look+1);
        G_row5 = G_row5+CX-(look+1);
        
        G_col1 = G_col1+CY-(look+1);
        G_col2 = G_col2+CY-(look+1);
        G_col3 = G_col3+CY-(look+1);
        G_col4 = G_col4+CY-(look+1);
        G_col5 = G_col5+CY-(look+1);
        
        
        for i = 1:length(G_row1)
            ParentX(G_row1(i),G_col1(i),CZ+2) = CX;
            ParentY(G_row1(i),G_col1(i),CZ+2) = CY;
            ParentZ(G_row1(i),G_col1(i),CZ+2) = CZ;
        end
        
        for i = 1:length(G_row2)
            ParentX(G_row2(i),G_col2(i),CZ+1) = CX;
            ParentY(G_row2(i),G_col2(i),CZ+1) = CY;
            ParentZ(G_row2(i),G_col2(i),CZ+1) = CZ;
        end
        
        for i = 1:length(G_row3)
            if G_row3(i)==CX && G_col3(i)==CY
                continue
            end
            ParentX(G_row3(i),G_col3(i),CZ) = CX;
            ParentY(G_row3(i),G_col3(i),CZ) = CY;
            ParentZ(G_row3(i),G_col3(i),CZ) = CZ;
        end
        
        for i = 1:length(G_row4)
            ParentX(G_row4(i),G_col4(i),CZ-1) = CX;
            ParentY(G_row4(i),G_col4(i),CZ-1) = CY;
            ParentZ(G_row4(i),G_col4(i),CZ-1) = CZ;
        end
        
        for i = 1:length(G_row5)
            ParentX(G_row5(i),G_col5(i),CZ-2) = CX;
            ParentY(G_row5(i),G_col5(i),CZ-2) = CY;
            ParentZ(G_row5(i),G_col5(i),CZ-2) = CZ;
        end
        
        
        
        
        if abs(Goal(1)-CX)<=(look-1) && abs(Goal(2)-CY)<=(look-1) && abs(Goal(3)-CZ)<=(look-1)
            REACHGOAL = 1;
            break
        end
        
    end
    
    
    % optimal = nan(128,3);
    if REACHGOAL
        optimal(1,:) = [Goal(1) Goal(2) Goal(3)];
        k=2;
        while 1
            CX_temp = int32(ParentX(CX,CY,CZ));
            CY_temp = int32(ParentY(CX,CY,CZ));
            CZ_temp = int32(ParentZ(CX,CY,CZ));
            
            CX = CX_temp;
            CY = CY_temp;
            CZ = CZ_temp;
            
            optimal(k,:) = [CX CY CZ];
            k = k+1;
            
            if CX==Start(1) && CY==Start(2) && CZ==Start(3)
                break
            end
        end
    end
    
end
start_point = [pos_init(1) pos_init(2) pos_init(3)];

% optimal_path_x = flip(single(((optimal(:,1)-start_point(1))-0.5) * 0.2 + 0.1));      % grid_size = 0.2
% optimal_path_y = flip(single(((optimal(:,2)-start_point(2))-0.5) * 0.2 + 0.1));
% optimal_path_z = flip(single(((optimal(:,3)-start_point(3))-0.5) * 0.2 + 0.1));
optimal_path_x = flip(single( (optimal(:,1)-start_point(1)) * 0.2 ));      % grid_size = 0.2
optimal_path_y = flip(single( (optimal(:,2)-start_point(2)) * 0.2 ));
optimal_path_z = flip(single( (optimal(:,3)-start_point(3)) * 0.2 ));


end

== matlab function waypoint_generation_ptCloud_200802_mapdata_filtering_8m_2/3D A* Algorithm/MATLAB Function8 ==
  data: octomap_center input; Obstacle output; pos_init input
function Obstacle = gen_3d_array(octomap_center,pos_init)

mapsize = [150 150 30];

Obstacle = int8(zeros(mapsize(1),mapsize(2),mapsize(3)));
grid_size = 0.2;
start_point = [pos_init(1) pos_init(2) pos_init(3)];

% align1 = int16(octomap_center/(grid_size)+0.5);
align1 = int16(octomap_center/(grid_size));
align2 = unique(align1,'rows');
align3 = [align2(:,1)+start_point(1) align2(:,2)+start_point(2) align2(:,3)+start_point(3)];

for i = 1:numel(align3)/3
    
    index_temp = align3(i,:);
    
    index_check = index_temp<3;
    if sum(index_check)>=1
        index_temp(index_check) = 3;
    end
    
    if index_temp(1) > mapsize(1)-2
        index_temp(1) = mapsize(1)-2;
    end
    if index_temp(2) > mapsize(2)-2
        index_temp(2) = mapsize(2)-2;
    end
    if index_temp(3) > mapsize(3)-2
        index_temp(3) = mapsize(3)-2;
    end
    

    index_x = index_temp(1)-1:index_temp(1)+1;
    index_y = index_temp(2)-1:index_temp(2)+1;
    index_z = index_temp(3)-1:index_temp(3)+1;

    Obstacle(index_x,index_temp(2)+1,index_temp(3)+1) = 1;
    Obstacle(index_x,index_temp(2)+1,index_temp(3)) = 1;
    Obstacle(index_x,index_temp(2)+1,index_temp(3)-1) = 1;
    Obstacle(index_x,index_temp(2),index_temp(3)+1) = 1;
    Obstacle(index_x,index_temp(2),index_temp(3)) = 1;
    Obstacle(index_x,index_temp(2),index_temp(3)-1) = 1;
    Obstacle(index_x,index_temp(2)-1,index_temp(3)+1) = 1;
    Obstacle(index_x,index_temp(2)-1,index_temp(3)) = 1;
    Obstacle(index_x,index_temp(2)-1,index_temp(3)-1) = 1;
    
%     Obstacle(index_temp(1)+1,index_temp(2)+2,index_z) = 1;
%     Obstacle(index_temp(1)+1,index_temp(2)-2,index_z) = 1;
%     Obstacle(index_temp(1)+1,index_y,index_temp(3)+2) = 1;
%     Obstacle(index_temp(1)+1,index_y,index_temp(3)-2) = 1;
%     Obstacle(index_temp(1),index_temp(2)+2,index_z) = 1;
%     Obstacle(index_temp(1),index_temp(2)-2,index_z) = 1;
%     Obstacle(index_temp(1),index_y,index_temp(3)+2) = 1;
%     Obstacle(index_temp(1),index_y,index_temp(3)-2) = 1;
%     Obstacle(index_temp(1)-1,index_temp(2)+2,index_z) = 1;
%     Obstacle(index_temp(1)-1,index_temp(2)-2,index_z) = 1;
%     Obstacle(index_temp(1)-1,index_y,index_temp(3)+2) = 1;
%     Obstacle(index_temp(1)-1,index_y,index_temp(3)-2) = 1;
    
    
    
    
%     Obstacle(index_temp(1)+2,index_temp(2)+2,index_z) = 1;
%     Obstacle(index_temp(1)+2,index_temp(2)+1,index_z) = 1;
%     Obstacle(index_temp(1)+2,index_temp(2),index_z) = 1;
%     Obstacle(index_temp(1)+2,index_temp(2)-1,index_z) = 1;
%     Obstacle(index_temp(1)+2,index_temp(2)-2,index_z) = 1;
%     
%     Obstacle(index_temp(1)+1,index_temp(2)+2,index_z) = 1;
%     Obstacle(index_temp(1)+1,index_temp(2)+1,index_z) = 1;
%     Obstacle(index_temp(1)+1,index_temp(2),index_z) = 1;
%     Obstacle(index_temp(1)+1,index_temp(2)-1,index_z) = 1;
%     Obstacle(index_temp(1)+1,index_temp(2)-2,index_z) = 1;
%     
%     Obstacle(index_temp(1),index_temp(2)+2,index_z) = 1;
%     Obstacle(index_temp(1),index_temp(2)+1,index_z) = 1;
%     Obstacle(index_temp(1),index_temp(2),index_z) = 1;
%     Obstacle(index_temp(1),index_temp(2)-1,index_z) = 1;
%     Obstacle(index_temp(1),index_temp(2)-2,index_z) = 1;
%     
%     Obstacle(index_temp(1)-1,index_temp(2)+2,index_z) = 1;
%     Obstacle(index_temp(1)-1,index_temp(2)+1,index_z) = 1;
%     Obstacle(index_temp(1)-1,index_temp(2),index_z) = 1;
%     Obstacle(index_temp(1)-1,index_temp(2)-1,index_z) = 1;
%     Obstacle(index_temp(1)-1,index_temp(2)-2,index_z) = 1;
%     
%     Obstacle(index_temp(1)-2,index_temp(2)+2,index_z) = 1;
%     Obstacle(index_temp(1)-2,index_temp(2)+1,index_z) = 1;
%     Obstacle(index_temp(1)-2,index_temp(2),index_z) = 1;
%     Obstacle(index_temp(1)-2,index_temp(2)-1,index_z) = 1;
%     Obstacle(index_temp(1)-2,index_temp(2)-2,index_z) = 1;
    
end

Obstacle(1:3,:,:)=1;
Obstacle(mapsize(1)-2:mapsize(1),:,:) = 1;
Obstacle(:,1:3,:) = 1;
Obstacle(:,mapsize(2)-2:mapsize(2),:) = 1;
Obstacle(:,:,1:3) = 1;
Obstacle(:,:,mapsize(3)-10:mapsize(3)) = 1;

end

== matlab function waypoint_generation_ptCloud_200802_mapdata_filtering_8m_2/Path Guidance/MATLAB Function ==
  data: X_vel_cmd output; Y_vel_cmd output; odom input; Z_vel_cmd output; optimal_path_x input size=[128 1]; optimal_path_y input size=[128 1]; optimal_path_z input size=[128 1]; yaw_cmd output
function [X_vel_cmd,Y_vel_cmd,Z_vel_cmd,yaw_cmd] = fcn(odom,optimal_path_x,optimal_path_y,optimal_path_z)

P_gain = 0.5;

path_length = length(optimal_path_x);
K = inf(path_length,1);
optimal_path_norm = inf(path_length,3);

% optimal_path_x_temp = optimal_path_x.Data';
% optimal_path_y_temp = optimal_path_y.Data';

optimal_path_norm(:,1) = single(optimal_path_x - odom(1));
optimal_path_norm(:,2) = single(optimal_path_y - odom(2));
optimal_path_norm(:,3) = single(optimal_path_z - odom(3));

% optimal_path = [optimal_path_x' optimal_path_y'];
% optimal_path_norm = optimal_path - [odom(1) odom(2)];

for i=1:path_length
    K(i) = norm(optimal_path_norm(i,:));
end

[~,m] = min(K);



% Z_cmd = optimal_path_z(m);
if m >= 128
    m = 127;
end
% Z_cmd = optimal_path_z(m+1) + APF_vector(3);         % prediction
% X_cmd = optimal_path_x(m+1) + APF_vector(1);
% Y_cmd = optimal_path_y(m+1) + APF_vector(2);
Z_cmd = optimal_path_z(m+1);       
X_cmd = optimal_path_x(m+1);
Y_cmd = optimal_path_y(m+1);

error_z = (Z_cmd - odom(3));
error_x = (X_cmd - odom(1));
error_y = (Y_cmd - odom(2));

Z_vel_cmd = double(error_z*P_gain);
X_vel_cmd = double(error_x*P_gain);
Y_vel_cmd = double(error_y*P_gain);
% yaw_cmd = atan2(Y_cmd-odom(2),X_cmd-odom(1));        % 고쳐야함 
% yaw_cmd = atan2(optimal_path_y(m+1)-odom(2),optimal_path_x(m+1)-odom(1)); 
if m <= 125
    yaw_vector1 = [optimal_path_x(m+1)-odom(1) optimal_path_y(m+1)-odom(2)] / norm([optimal_path_x(m+1)-odom(1) optimal_path_y(m+1)-odom(2)]);
    yaw_vector2 = [optimal_path_x(m+2)-odom(1) optimal_path_y(m+2)-odom(2)] / norm([optimal_path_x(m+2)-odom(1) optimal_path_y(m+2)-odom(2)]);
    yaw_vector3 = [optimal_path_x(m+3)-odom(1) optimal_path_y(m+3)-odom(2)] / norm([optimal_path_x(m+3)-odom(1) optimal_path_y(m+3)-odom(2)]);
    yaw_vector = yaw_vector1 + yaw_vector2 + yaw_vector3;
    yaw_cmd = double( atan2(yaw_vector(2),yaw_vector(1)) );
%     yaw_cmd = double( ( atan2(optimal_path_y(m+1)-odom(2),optimal_path_x(m+1)-odom(1)) + atan2(optimal_path_y(m+2)-odom(2),optimal_path_x(m+2)-odom(1)) + atan2(optimal_path_y(m+3)-odom(2),optimal_path_x(m+3)-odom(1)) ) / 3 );
else
    yaw_cmd = 0;
end

end

== matlab function waypoint_generation_ptCloud_200802_mapdata_filtering_8m_2/Motor_Dynamics/Motor Dynamics/Motor Rotation Speed Generation ==
  data: w_dot_cmd input; w_state input; w_motor output; T_require output; Moment output; w_motor_square output; a_cmd input; DCM input
function [w_motor,T_require,Moment,w_motor_square] = fcn(w_dot_cmd,w_state,a_cmd,DCM)

w_motor        = zeros(4,1);
% ============= Quadrotor Spec  ==========================================%
kafa_f = 6.41*10^-6;                    % thrust coefficient
kafa_tau = 1.69*10^-2;                  % moment coefficient

L = 0.22/2;                               % length ( motor to motor) [m]
M = 0.5 ; %mass    [Kg]

I_T = [3.2*10^-3,3.2*10^-3,5.5*10^-3];  % total moment
I_P = [0,0,1.5*10^-5];                  % propeller reaction moment
I_B = I_T - 4*I_P;                      % frame inertia moment
Inertia = diag(I_B);
% 
% T_require = M * norm(a_cmd);
T_hover = [0,0,1]; %Thrust
R_z = DCM(:,3);
g = 9.8; %gravity [m/s^2]
T_require = M*(abs(a_cmd) / dot(T_hover,R_z));


Moment = Inertia*w_dot_cmd + cross(w_state,Inertia*w_state);

A = [1       ,  1         ,   1         ,   1;
    0        ,  L         ,   0         ,  -L;
    -L       ,  0         ,   L         ,   0;
    kafa_tau , -kafa_tau  ,   kafa_tau  ,  -kafa_tau];

w_motor_square = A^-1 * [T_require;Moment]/kafa_f;

for i = 1:length(w_motor_square)
    w_motor(i) = sqrt(abs(w_motor_square(i)));
end

== matlab function waypoint_generation_ptCloud_200802_mapdata_filtering_8m_2/Quadrotor Dynamics/중력항 고려 ==
  data: Mg input; DCM_e2b input; Fe output
function Fe = fcn(Mg,DCM_e2b)

Fe=DCM_e2b*Mg;

== matlab function waypoint_generation_ptCloud_200802_mapdata_filtering_8m_2/Generation_Angle_error/Attitude Generation(psi^*) ==
  data: R_rp_x input; acc_cmd input; Bearing_angle input; psi_angle_error output
function psi_angle_error   = fcn(R_rp_x,acc_cmd,Bearing_angle)
%#codegen

acc_cmd_unit  = acc_cmd / norm(acc_cmd); % define hat(k)_B_des
sigma = Bearing_angle;

j_sigma_des = [-sin(sigma),cos(sigma),0]; % hat(i)_sigma_des

i_B_des =  cross(j_sigma_des,acc_cmd_unit);
R_sp_x  =  i_B_des;
% 
% temp  = cross(R_rp_x,R_sp_x);
% temp2 = dot(R_rp_x,R_sp_x);

psi_angle_error = atan(cross(R_rp_x,R_sp_x)*acc_cmd_unit/dot(R_rp_x,R_sp_x))*acc_cmd_unit(3)^2;

% psi_angle_error = atan(norm(cross(R_rp_x,R_sp_x))/dot(R_rp_x,R_sp_x));

== matlab function waypoint_generation_ptCloud_200802_mapdata_filtering_8m_2/Generation_Angle_error/Attitude Generation(phi,theta,psi^*) ==
  data: angle_error input; psi_angle_error input; angle_error_result output
function angle_error_result  = fcn(angle_error,psi_angle_error)
%#codegen

angle_error_result = [angle_error(1);angle_error(2);psi_angle_error];

% if norm(temp) ~= 0
%     angle_error_result  = temp / norm(temp);
% else
%     angle_error_result  = temp;
% end
